simulink model "diagrama4"  (R2014a)
settings: Solver=ode45  StartTime=0.0  StopTime=10  FixedStep=1e-3  RelTol=1e-3
values from neighbouring files (symbols this model uses):
  G = lqr(A,B,Q,R)    [projeto.m]
  Phi_i = pi/6    (= 0.523598775598)    [projeto.m]
undefined symbols (not defined in the file or in its folder): magnitude, opt
libraries: simulink x6
settings Model: Creator=fabrizio  LastModifiedBy=user
settings DataIOCC: Refine=10

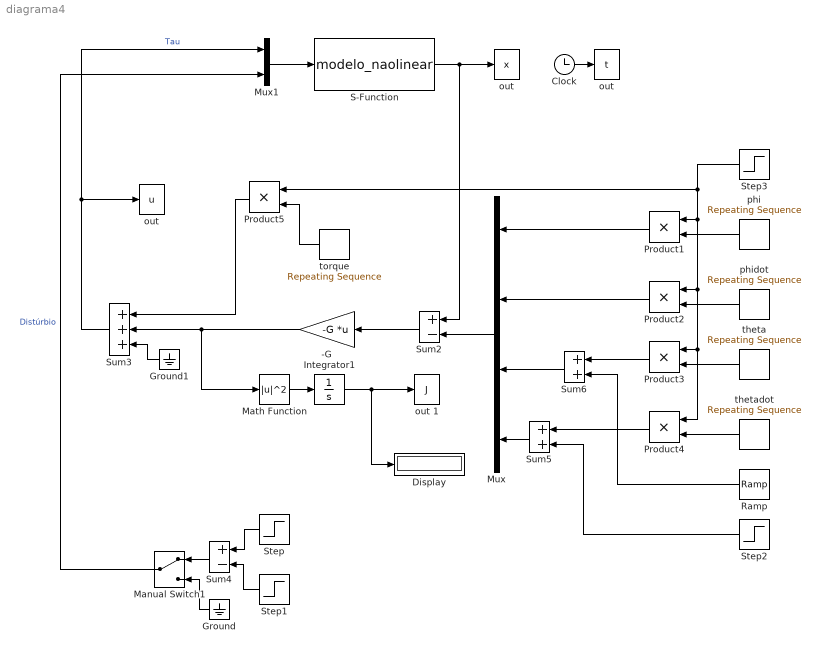
== system diagrama4 ==
  -G : Gain  Gain=-G  Multiplication=Matrix(K*u)
  Clock : Clock
  Display : Display
  Ground : Ground
  Ground1 : Ground
  Integrator1 : Integrator  InitialCondition="[  0   0   0   0  ]"
  Manual Switch1 : ManualSwitch
  Math Function : Math  Operator=magnitude^2  SaturateOnIntegerOverflow=on
  Mux : Mux
  Mux1 : Mux  Inputs=2
  Product{1..5} (5 alike) : Product
  Ramp : simulink/Sources/Ramp  slope=1  start=opt.ti(end)+1  X0=0
  S-Function : S-Function  FunctionName=modelo_naolinear  Parameters="[  Phi_i   0   0   0  ]'"  EnableBusSupport=off
  Step : Step  Time=10  After=-2  SampleTime=0
  Step1 : Step  Time=10.1  After=-2  SampleTime=0
  Step2 : Step  Time=opt.ti(end)+1  SampleTime=0
  Step3 : Step  Time=opt.ti(end)  Before=1  After=0  SampleTime=0
  Sum2 : Sum  Inputs=+-
  Sum3 : Sum  Inputs=+++
  Sum4 : Sum  Inputs=+-
  Sum5 : Sum
  Sum6 : Sum
  out : ToWorkspace  VariableName=t  SampleTime=-1
  "out " : ToWorkspace  VariableName=x  SampleTime=-1
  "out  " : ToWorkspace  VariableName=u  SampleTime=-1
  out 1 : ToWorkspace  VariableName=J  SampleTime=-1
  phi : simulink/Sources/Repeating Sequence  rep_seq_t=[ opt.ti ]  rep_seq_y=[ opt.phi ]
  phidot : simulink/Sources/Repeating Sequence  rep_seq_t="[ opt.ti  ]"  rep_seq_y=[ opt.phid ]
  theta : simulink/Sources/Repeating Sequence  rep_seq_t="[ opt.ti  ]"  rep_seq_y=[opt.theta ]
  thetadot : simulink/Sources/Repeating Sequence  rep_seq_t=[ opt.ti ]  rep_seq_y=[ opt.thetad ]
  torque : simulink/Sources/Repeating Sequence  rep_seq_t=[0; opt.tc ]  rep_seq_y=[ opt.tau ; opt.tau(end) ]
  wires:
  Sum2/1 -> -G/1
  Clock/1 -> out/1
  Mux/1 -> Sum2/2
  Math Function/1 -> Integrator1/1
  Sum3/1 -> Mux1/1, "out  "/1  "Tau"
  -G/1 -> Sum3/2, Math Function/1
  Product1/1 -> Mux/1
  Product2/1 -> Mux/2
  phi/1 -> Product1/2
  phidot/1 -> Product2/2
  theta/1 -> Product3/2
  thetadot/1 -> Product4/2
  Step3/1 -> Product4/1, Product3/1, Product2/1, Product1/1, Product5/1
  Product5/1 -> Sum3/1
  torque/1 -> Product5/2
  Sum5/1 -> Mux/4
  Product4/1 -> Sum5/1
  Sum6/1 -> Mux/3
  Product3/1 -> Sum6/1
  Ramp/1 -> Sum6/2
  Step2/1 -> Sum5/2
  Integrator1/1 -> Display/1, out 1/1
  S-Function/1 -> Sum2/1, "out "/1
  Step/1 -> Sum4/1
  Step1/1 -> Sum4/2
  Sum4/1 -> Manual Switch1/1
  Ground/1 -> Manual Switch1/2
  Manual Switch1/1 -> Mux1/2  "Distúrbio"
  Mux1/1 -> S-Function/1
  Ground1/1 -> Sum3/3
